simulink model "ex5_p2_PREDATION"  (Simulink 7.9)
settings: Solver=ode45  StartTime=0.0  StopTime=40.0  RelTol=1e-3
libraries: simulink x1
settings Model: Creator=bazkoale  LastModifiedBy=alex
settings DataIOCC: SignalLoggingSaveFormat=Dataset
settings OptimizationCC: ExpressionDepthLimit=128
settings DebuggingCC: MultiTaskDSMMsg=warning  MultiTaskCondExecSysMsg=none  StrictBusMsg=None
settings RTWCC: IncludeERTFirstTime=on
settings CodeAppCC: CustomSymbolStrType=$N$R$M_T

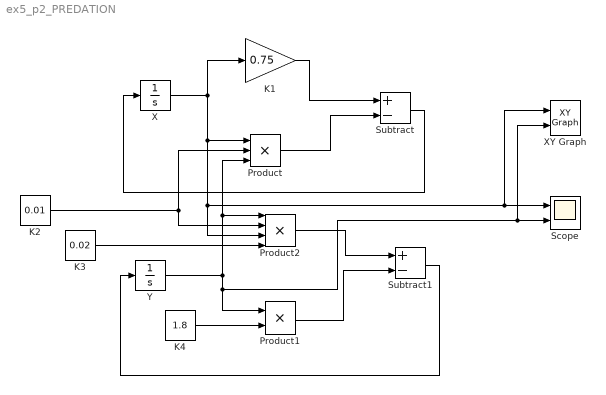
== system ex5_p2_PREDATION ==
  K1 : Gain  Gain=0.75
  K2 : Constant  Value=0.01
  K3 : Constant  Value=0.02
  K4 : Constant  Value=1.8
  Product : Product  Inputs=3
  Product1 : Product
  Product2 : Product  Inputs=4
  Scope : Scope  NumInputPorts=2
      settings: YMin=-5~-5  YMax=5~5
  Subtract : Sum  Inputs=+-
  Subtract1 : Sum  Inputs=+-
  X : Integrator  InitialCondition=140000
  XY Graph : simulink/Sinks/XY Graph  xmin=0  xmax=150000  ymin=0  ymax=3000  st=-1
  Y : Integrator  InitialCondition=10
  wires:
  K1/1 -> Subtract/1
  Subtract/1 -> X/1
  K2/1 -> Product2/2, Product/2
  Product2/1 -> Subtract1/1
  Subtract1/1 -> Y/1
  K4/1 -> Product1/2
  Product1/1 -> Subtract1/2
  Product/1 -> Subtract/2
  K3/1 -> Product2/4
  X/1 -> XY Graph/1, Scope/1, Product2/3, Product/1, K1/1
  Y/1 -> Product2/1, Product/3, Product1/1, XY Graph/2, Scope/2
